simulink model "FIVELEVEL"  (R2017a)
settings: Solver=ode23tb  StartTime=0.0  StopTime=.2  FixedStep=1e-6  MaxStep=1e-4  RelTol=1e-3
libraries: powerlib x16, simulink x1
settings Model: Creator=acer  LastModifiedBy=acer
settings SolverCC: ZeroCrossAlgorithm=Adaptive  SolverResetMethod=Robust

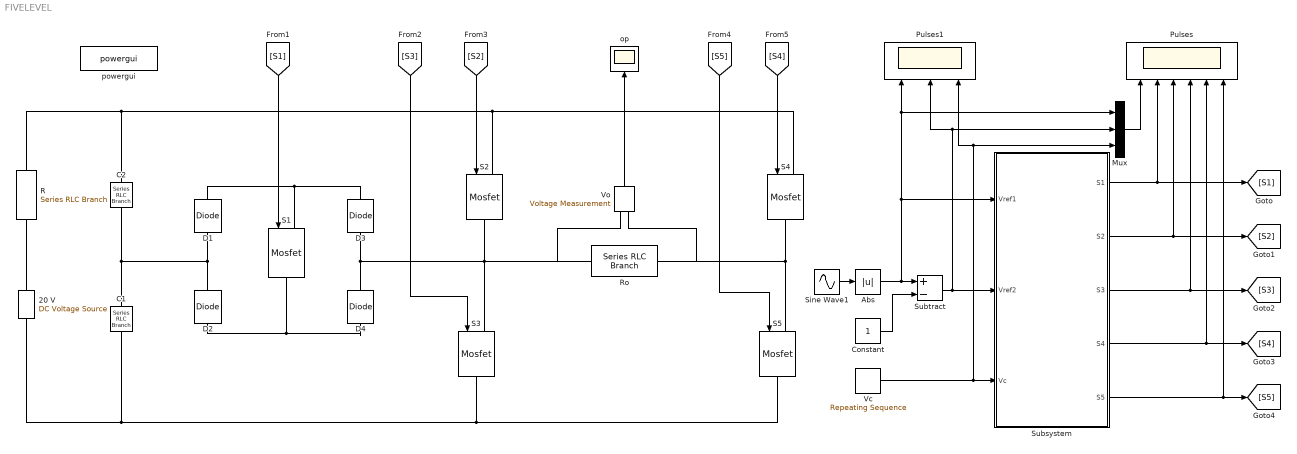
== system FIVELEVEL ==
  20 V : powerlib/Electrical Sources/DC Voltage Source  Amplitude=20  Measurements=None
  Abs : Abs
  C1 : powerlib/Elements/Series RLC Branch  LConnTagsString=__new0  RConnTagsString=__new0  BranchType=C  Resistance=100  Inductance=1e-3  SetiL0=off  InitialCurrent=0  Capacitance=2  Setx0=on  InitialVoltage=10  Measurements=None
  C2 : powerlib/Elements/Series RLC Branch  LConnTagsString=__new0  RConnTagsString=__new0  BranchType=C  Resistance=100  Inductance=1e-3  SetiL0=off  InitialCurrent=0  Capacitance=2  Setx0=on  InitialVoltage=10  Measurements=None
  Constant : Constant
  D{1..4} (4 alike) : powerlib/Power Electronics/Diode  Ron=0.001  Lon=0  Vf=.05  IC=0  UseSnubber=off  Rs=500  Cs=250e-9  Measurements=off
  Mux : Mux  Inputs=3
  Pulses : Scope  NumInputPorts=6
  Pulses1 : Scope  NumInputPorts=3
  R : powerlib/Elements/Series RLC Branch  LConnTagsString=__new0  RConnTagsString=__new0  BranchType=R  Resistance=1e-8  Inductance=1e-3  SetiL0=off  InitialCurrent=0  Capacitance=1e-6  Setx0=off  InitialVoltage=0  Measurements=None
  Ro : powerlib/Elements/Series RLC Branch  LConnTagsString=__new0  RConnTagsString=__new0  BranchType=R  Resistance=20  Inductance=1e-3  SetiL0=off  InitialCurrent=0  Capacitance=1e-6  Setx0=off  InitialVoltage=0  Measurements=None
  S{1..5} (5 alike) : powerlib/Power Electronics/Mosfet  Ron=0.1  Lon=0  Rd=0.01  Vfd=0  IC=0  Rs=1e5  Cs=inf  Measurements=off
  Sine Wave1 : Sin  Amplitude=2.5  Frequency=2*pi*50  SampleTime=0  VectorParams1D=off
  Subsystem : Subsystem
  Subtract : Sum  Inputs=+-
  Vc : simulink/Sources/Repeating Sequence  rep_seq_t="[0  1e-5 2e-5]"  rep_seq_y=[0 1 0]
  Vo : powerlib/Measurements/Voltage Measurement  PhasorSimulation=off  OutputType=Complex  PSBequivalent=0
  op : Scope
  powergui : powerlib/powergui  Priority=1  SimulationMode=Continuous  SampleTime=1e-6  frequency=60  Iterations=50  frequencyindice=0  Pbase=100e6  ErrMax=1e-4  UnitsV=kV  UnitsW=MW  buscounter=0  FunctionMessages=off  echomessages=off  EnableUseOfTLC=off  CurrentSourceSwitches=off  DisableSnubberDevices=off  DisableRonSwitches=off  DisableVfSwitches=off  DisplayEquations=off  SolverType=Tustin/Backward Euler (TBE)  Interpol=off  ExternalGateDelay=off  methode=off  Ts=100  x0status=blocks  SPID=off  SwTol=0  HookPort=off  RestoreLinks=warning  ResistiveCurrentMeasurement=off  Frange=[0:2:500]  Ylog=off  Xlog=on  ShowGrid=off  save=off  variable=ZData  structure=outputVoltage  ZoomFFT=off  StartTime=0  cycles=10  DisplayStyle=3  fundamental=50  FreqAxis=off  MaxFrequency=1000  frequencyindicesteady=1  RmsSteady=1  display=off
  wires:
  [S1] -> S1/1
  [S2] -> S2/1
  [S3] -> S3/1
  [S4] -> S4/1
  [S5] -> S5/1
  Vo/1 -> op/1
  Sine Wave1/1 -> Abs/1
  Subtract/1 -> Subsystem/2(Vref2), Pulses1/2, Mux/2
  Constant/1 -> Subtract/2
  Subsystem/1(S1) -> [S1], Pulses/2
  Subsystem/3(S3) -> [S3], Pulses/4
  Subsystem/4(S4) -> [S4], Pulses/5
  Vc/1 -> Subsystem/3(Vc), Pulses1/3, Mux/3
  Mux/1 -> Pulses/1
  Subsystem/2(S2) -> [S2], Pulses/3
  Abs/1 -> Mux/1, Pulses1/1, Subsystem/1(Vref1), Subtract/1
  Subsystem/5(S5) -> [S5], Pulses/6
  connections:
  D1/RConn1 -- S1/LConn1 -- D3/RConn1
  D4/LConn1 -- S1/RConn1 -- D2/LConn1
  C1/LConn1 -- C2/RConn1 -- D2/RConn1 -- D1/LConn1
  D3/LConn1 -- Vo/LConn1 -- Ro/LConn1 -- S2/RConn1 -- S3/LConn1 -- D4/RConn1
  S2/LConn1 -- S4/LConn1 -- R/RConn1 -- C2/LConn1
  S3/RConn1 -- S5/RConn1 -- C1/RConn1 -- 20 V/LConn1
  S4/RConn1 -- Vo/LConn2 -- Ro/RConn1 -- S5/LConn1
  R/LConn1 -- 20 V/RConn1

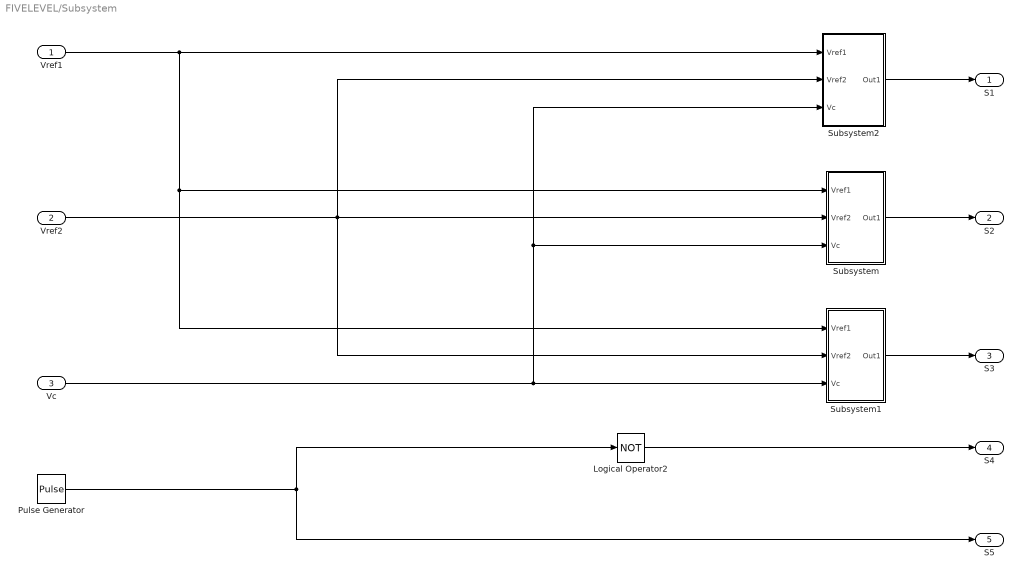
== system FIVELEVEL/Subsystem ==
  Vref1 : Inport
  Vref2 : Inport  Port=2
  Vc : Inport  Port=3
  Logical Operator2 : Logic  Operator=NOT  AllPortsSameDT=off  OutDataTypeStr=boolean
  Pulse Generator : DiscretePulseGenerator  PulseType=Time based  Period=.02  PulseWidth=50
  Subsystem : Subsystem
  Subsystem1 : Subsystem
  Subsystem2 : Subsystem
  S1 : Outport
  S2 : Outport  Port=2
  S3 : Outport  Port=3
  S4 : Outport  Port=4
  S5 : Outport  Port=5
  wires:
  Subsystem1/1(Out1) -> S3/1
  Pulse Generator/1 -> Logical Operator2/1, S5/1
  Logical Operator2/1 -> S4/1
  Subsystem/1(Out1) -> S2/1
  Subsystem2/1(Out1) -> S1/1
  Vref1/1 -> Subsystem1/1(Vref1), Subsystem/1(Vref1), Subsystem2/1(Vref1)
  Vref2/1 -> Subsystem2/2(Vref2), Subsystem1/2(Vref2), Subsystem/2(Vref2)
  Vc/1 -> Subsystem2/3(Vc), Subsystem/3(Vc), Subsystem1/3(Vc)

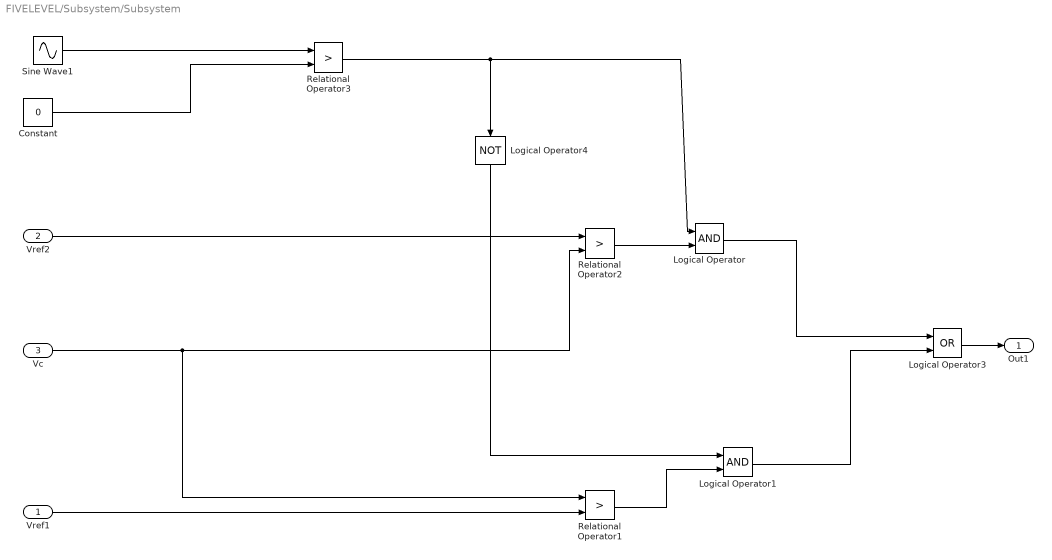
== system FIVELEVEL/Subsystem/Subsystem ==
  Vref1 : Inport
  Vref2 : Inport  Port=2
  Vc : Inport  Port=3
  Constant : Constant  Value=0
  Logical Operator : Logic  AllPortsSameDT=off  OutDataTypeStr=boolean
  Logical Operator1 : Logic  AllPortsSameDT=off  OutDataTypeStr=boolean
  Logical Operator3 : Logic  Operator=OR  AllPortsSameDT=off  OutDataTypeStr=boolean
  Logical Operator4 : Logic  Operator=NOT  AllPortsSameDT=off  OutDataTypeStr=boolean
  Relational Operator1 : RelationalOperator  Operator=>  OutDataTypeStr=boolean  RndMeth=Nearest
  Relational Operator2 : RelationalOperator  Operator=>  OutDataTypeStr=boolean  RndMeth=Nearest
  Relational Operator3 : RelationalOperator  Operator=>  OutDataTypeStr=boolean  RndMeth=Nearest
  Sine Wave1 : Sin  Amplitude=100  Frequency=2*pi*50  SampleTime=0  VectorParams1D=off
  Out1 : Outport
  wires:
  Vref1/1 -> Relational Operator1/2
  Vref2/1 -> Relational Operator2/1
  Vc/1 -> Relational Operator1/1, Relational Operator2/2
  Relational Operator2/1 -> Logical Operator/2
  Logical Operator4/1 -> Logical Operator1/1
  Relational Operator1/1 -> Logical Operator1/2
  Logical Operator/1 -> Logical Operator3/1
  Logical Operator1/1 -> Logical Operator3/2
  Logical Operator3/1 -> Out1/1
  Sine Wave1/1 -> Relational Operator3/1
  Constant/1 -> Relational Operator3/2
  Relational Operator3/1 -> Logical Operator/1, Logical Operator4/1

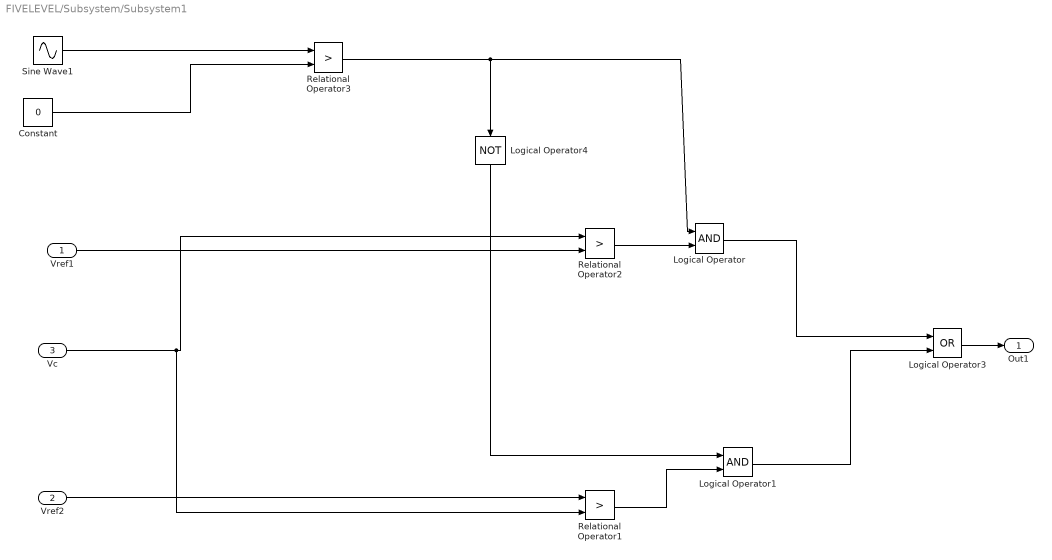
== system FIVELEVEL/Subsystem/Subsystem1 ==
  Vref1 : Inport
  Vref2 : Inport  Port=2
  Vc : Inport  Port=3
  Constant : Constant  Value=0
  Logical Operator : Logic  AllPortsSameDT=off  OutDataTypeStr=boolean
  Logical Operator1 : Logic  AllPortsSameDT=off  OutDataTypeStr=boolean
  Logical Operator3 : Logic  Operator=OR  AllPortsSameDT=off  OutDataTypeStr=boolean
  Logical Operator4 : Logic  Operator=NOT  AllPortsSameDT=off  OutDataTypeStr=boolean
  Relational Operator1 : RelationalOperator  Operator=>  OutDataTypeStr=boolean  RndMeth=Nearest
  Relational Operator2 : RelationalOperator  Operator=>  OutDataTypeStr=boolean  RndMeth=Nearest
  Relational Operator3 : RelationalOperator  Operator=>  OutDataTypeStr=boolean  RndMeth=Nearest
  Sine Wave1 : Sin  Amplitude=100  Frequency=2*pi*50  SampleTime=0  VectorParams1D=off
  Out1 : Outport
  wires:
  Vref1/1 -> Relational Operator2/2
  Vc/1 -> Relational Operator1/2, Relational Operator2/1
  Relational Operator2/1 -> Logical Operator/2
  Logical Operator4/1 -> Logical Operator1/1
  Relational Operator1/1 -> Logical Operator1/2
  Logical Operator/1 -> Logical Operator3/1
  Logical Operator1/1 -> Logical Operator3/2
  Logical Operator3/1 -> Out1/1
  Sine Wave1/1 -> Relational Operator3/1
  Constant/1 -> Relational Operator3/2
  Relational Operator3/1 -> Logical Operator/1, Logical Operator4/1
  Vref2/1 -> Relational Operator1/1

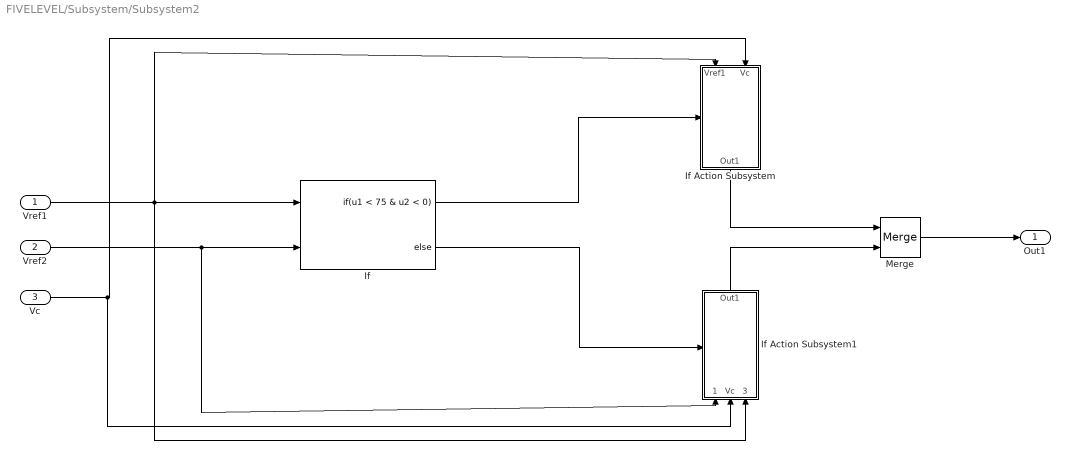
== system FIVELEVEL/Subsystem/Subsystem2 ==
  Vref1 : Inport
  Vref2 : Inport  Port=2
  Vc : Inport  Port=3
  If : If  NumInputs=2  IfExpression=u1 < 75 & u2 < 0
  If Action Subsystem : Subsystem  TreatAsAtomicUnit=on
  If Action Subsystem1 : Subsystem  TreatAsAtomicUnit=on
  Merge : Merge
  Out1 : Outport
  wires:
  Vref1/1 -> If Action Subsystem1/3(Vref1), If/1, If Action Subsystem/1(Vref1)
  Merge/1 -> Out1/1
  Vref2/1 -> If Action Subsystem1/1(Vref2), If/2
  If/2 -> If Action Subsystem1/Action
  If/1 -> If Action Subsystem/Action
  If Action Subsystem/1(Out1) -> Merge/1
  If Action Subsystem1/1(Out1) -> Merge/2
  Vc/1 -> If Action Subsystem1/2(Vc), If Action Subsystem/2(Vc)

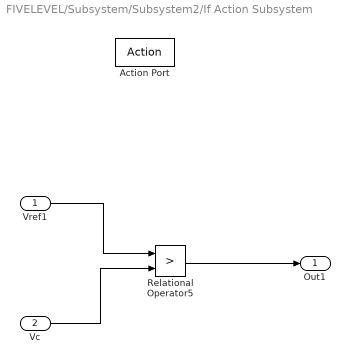
== system FIVELEVEL/Subsystem/Subsystem2/If Action Subsystem ==
  Vref1 : Inport
  Vc : Inport  Port=2
  Action Port : ActionPort  ActionType=then
  Relational Operator5 : RelationalOperator  Operator=>  OutDataTypeStr=boolean  RndMeth=Nearest
  Out1 : Outport
  wires:
  Vref1/1 -> Relational Operator5/1
  Vc/1 -> Relational Operator5/2
  Relational Operator5/1 -> Out1/1

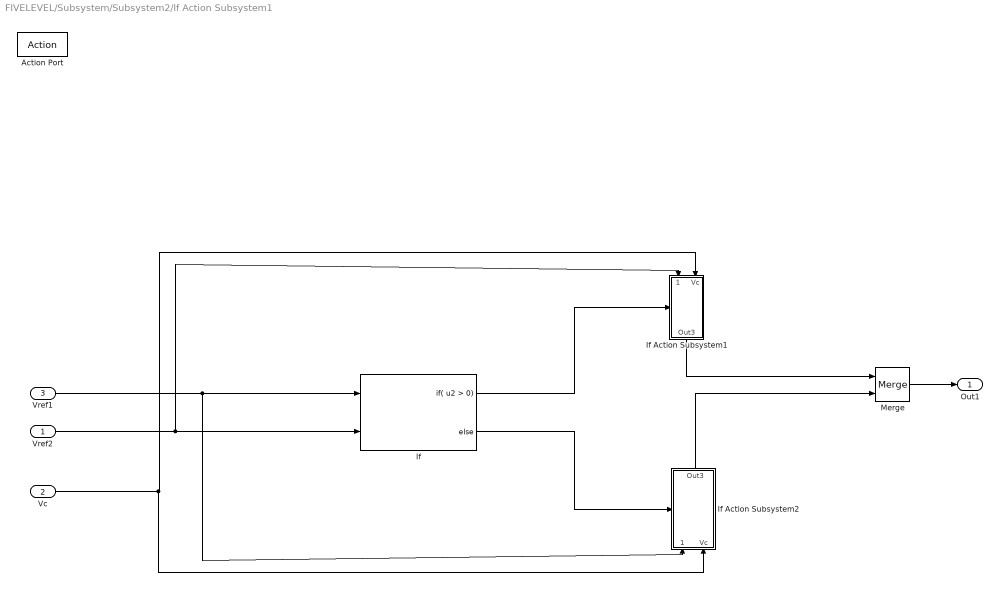
== system FIVELEVEL/Subsystem/Subsystem2/If Action Subsystem1 ==
  Vref2 : Inport
  Vc : Inport  Port=2
  Vref1 : Inport  Port=3
  Action Port : ActionPort  ActionType=else
  If : If  NumInputs=2  IfExpression=u2 > 0
  If Action Subsystem1 : Subsystem  TreatAsAtomicUnit=on
  If Action Subsystem2 : Subsystem  TreatAsAtomicUnit=on
  Merge : Merge
  Out1 : Outport
  wires:
  Vref1/1 -> If Action Subsystem2/1(Vref1), If/1
  Vref2/1 -> If Action Subsystem1/1(Vref2), If/2
  If/1 -> If Action Subsystem1/Action
  If/2 -> If Action Subsystem2/Action
  If Action Subsystem1/1(Out3) -> Merge/1
  If Action Subsystem2/1(Out3) -> Merge/2
  Merge/1 -> Out1/1
  Vc/1 -> If Action Subsystem2/2(Vc), If Action Subsystem1/2(Vc)

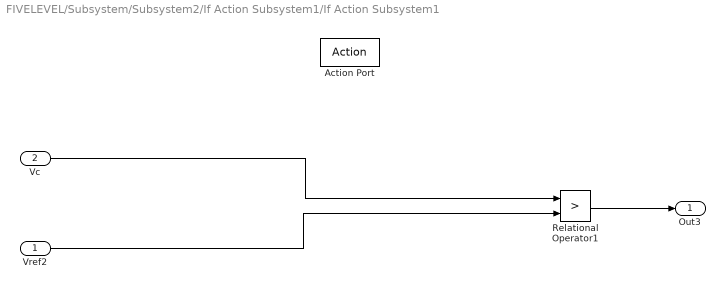
== system FIVELEVEL/Subsystem/Subsystem2/If Action Subsystem1/If Action Subsystem1 ==
  Vref2 : Inport
  Vc : Inport  Port=2
  Action Port : ActionPort  ActionType=then
  Relational Operator1 : RelationalOperator  Operator=>  OutDataTypeStr=boolean  RndMeth=Nearest
  Out3 : Outport
  wires:
  Relational Operator1/1 -> Out3/1
  Vc/1 -> Relational Operator1/1
  Vref2/1 -> Relational Operator1/2

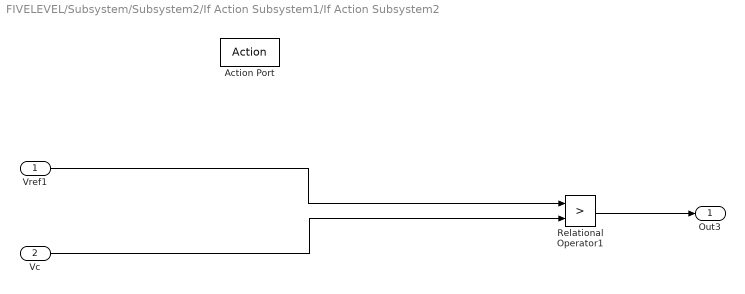
== system FIVELEVEL/Subsystem/Subsystem2/If Action Subsystem1/If Action Subsystem2 ==
  Vref1 : Inport
  Vc : Inport  Port=2
  Action Port : ActionPort  ActionType=else
  Relational Operator1 : RelationalOperator  Operator=>  OutDataTypeStr=boolean  RndMeth=Nearest
  Out3 : Outport
  wires:
  Relational Operator1/1 -> Out3/1
  Vref1/1 -> Relational Operator1/1
  Vc/1 -> Relational Operator1/2
